simulink model "model_p5"  (R2020b)
settings: Solver=VariableStepAuto  StartTime=0.0  StopTime=10.0  RelTol=1e-3
settings Model: Creator=ADMIN  LastModifiedBy=ADMIN

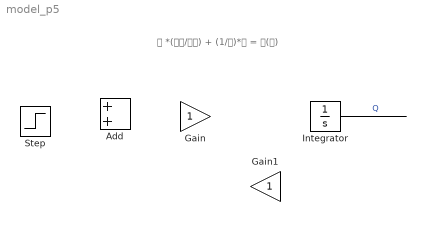
== system model_p5 ==
  note: 𝑅 *(𝑑𝑄/𝑑𝑡) + (1/𝐶)*𝑄 = 𝐸(𝑡)
  Add : Sum
  Gain : Gain
  Gain1 : Gain
  Integrator : Integrator
  Step : Step  SampleTime=0
  wires:
  Integrator/1 -> ?  "Q"
  ? -> Integrator/1  "Q_dot"
